simulink subsystem "classification_bnp_score"  (R2019b)
settings: Solver=VariableStepAuto  StartTime=0.0  StopTime=10.0  RelTol=1e-3
settings Model: Creator=RH  LastModifiedBy=RH

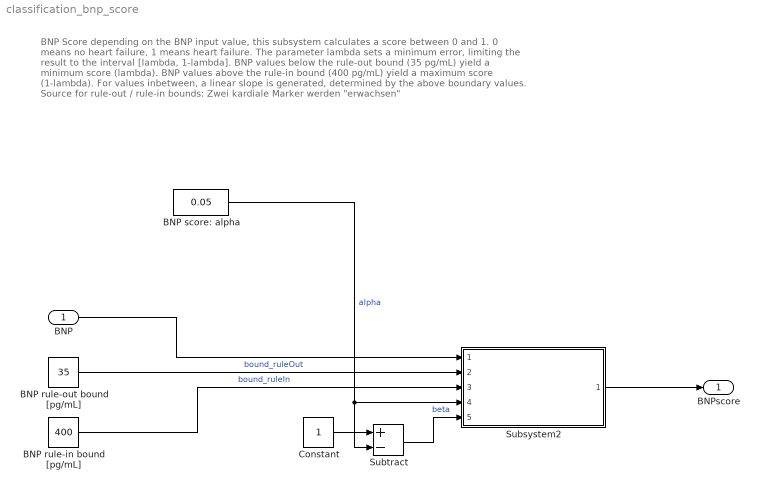
== system classification_bnp_score ==
  note: BNP Score
      | depending on the BNP input value, this subsystem calculates a score between 0 and 1.
      | 0 means no heart failure, 1 means heart failure.
      | The parameter lambda sets a minimum error, limiting the result to the interval [lambda, 1-lambda].
      | BNP values below the rule-out bound (35 pg/mL) yield a minimum score (lambda).
      | BNP values above the rule-in bound (400 pg/mL) yield a maximum score (1-lambda).
      | For values inbetween, a linear slope is generated, determined by the above boundary values.
      |
      | Source for rule-out / rule-in bounds: Zwei kardiale Marker werden "erwachsen"
  BNP : Inport  Unit=pg/mL
  BNP rule-in bound [pg/mL] : Constant  Value=400
  BNP rule-out bound [pg/mL] : Constant  Value=35
  BNP score: alpha : Constant  Value=0.05
  Constant : Constant
  Subsystem2 : Subsystem  ReferencedSubsystem=linear_slope_score
  Subtract : Sum  Inputs=+-
  BNPscore : Outport  Unit=1
  wires:
  BNP score: alpha/1 -> Subtract/2, Subsystem2/4  "alpha"
  Constant/1 -> Subtract/1
  Subtract/1 -> Subsystem2/5  "beta"
  BNP/1 -> Subsystem2/1
  BNP rule-out bound [pg/mL]/1 -> Subsystem2/2  "bound_ruleOut"
  BNP rule-in bound [pg/mL]/1 -> Subsystem2/3  "bound_ruleIn"
  Subsystem2/1 -> BNPscore/1
